simulink model "test_simple"  (R2015a)
settings: Solver=ode45  StartTime=0.0  StopTime=inf  RelTol=1e-3
libraries: CrazyFlie_lib x1
settings Model: Creator=rshum  LastModifiedBy=rshum

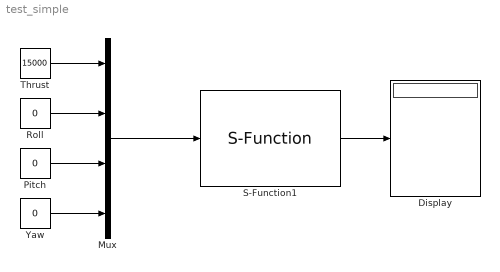
== system test_simple ==
  Display : Display
  Mux : Mux
  Pitch : Constant  Value=0
  Roll : Constant  Value=0
  S-Function1 : CrazyFlie_lib/S-Function
  Thrust : Constant  Value=15000
  Yaw : Constant  Value=0
  wires:
  Mux/1 -> S-Function1/1
  Thrust/1 -> Mux/1
  Roll/1 -> Mux/2
  Pitch/1 -> Mux/3
  Yaw/1 -> Mux/4
  S-Function1/1 -> Display/1
